simulink model "B1c"  (R2018a)
settings: Solver=VariableStepAuto  StartTime=0.0  StopTime=10  RelTol=1e-3
settings Model: Creator=daniel  LastModifiedBy=daniel

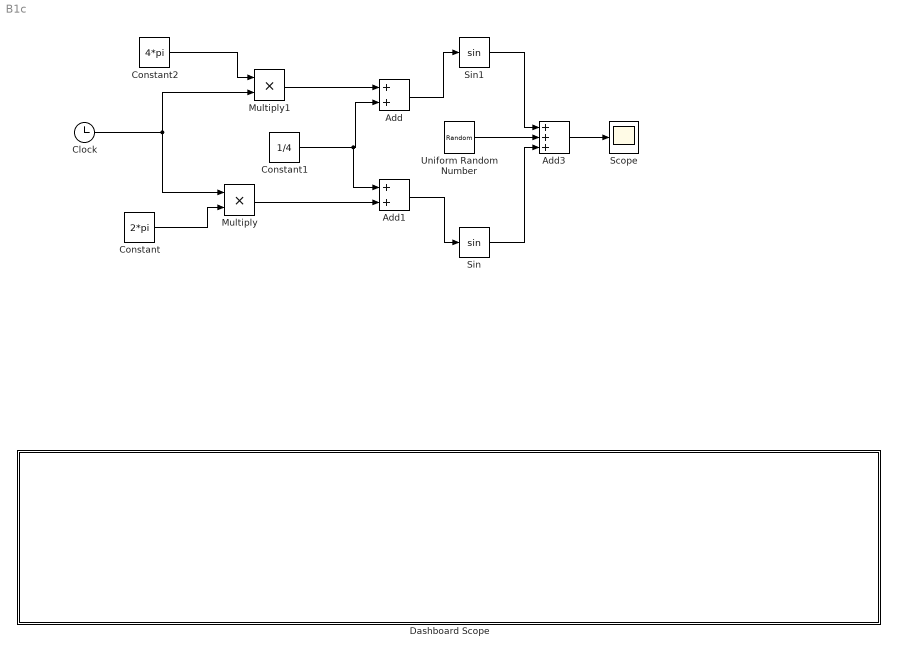
== system B1c ==
  Add : Sum
  Add1 : Sum
  Add3 : Sum  Inputs=3
  Clock : Clock
  Constant : Constant  Value=2*pi
  Constant1 : Constant  Value=1/4
  Constant2 : Constant  Value=4*pi
  Dashboard Scope : Subsystem  DialogController=hmiCreateDDGDialog  IsWebBlock=on  mask(MWDashboardBlock){webBlockId=babae165-9618-460c-bd61-f7bc25b1f03f, webBlockType=sdiscope, ShowInitialText=on, HMISrcModelName=B1c}
      mask prompts: webBlockId "WebBlock Id"; webBlockType "WebBlock Type"; HMISrcModelName "Source Model"
      mask help: SimulinkHMI:dialogs:HMIScopeDialogDesc
      mask Help: helpview([docroot '/mapfiles/simulink.map'], 'hmi_scope')
      mask Display:
      | if strcmp(get_param(bdroot(gcb),'BlockDiagramType'), 'library')
      |     image([(matlabroot) '/toolbox/simulink/hmi/icons/DashboardScope.png']);
      | end
  Multiply : Product
  Multiply1 : Product
  Scope : Scope
  Sin : Trigonometry
  Sin1 : Trigonometry
  Uniform Random Number : UniformRandomNumber  Minimum=-0.5  Maximum=0.5  Seed=13  SampleTime=0.1
  wires:
  Constant/1 -> Multiply/2
  Add1/1 -> Sin/1
  Clock/1 -> Multiply/1, Multiply1/2
  Constant2/1 -> Multiply1/1
  Multiply1/1 -> Add/1
  Multiply/1 -> Add1/2
  Constant1/1 -> Add/2, Add1/1
  Add/1 -> Sin1/1
  Sin1/1 -> Add3/1
  Sin/1 -> Add3/3
  Add3/1 -> Scope/1
  Uniform Random Number/1 -> Add3/2

== system B1c/Dashboard Scope ==
